simulink model "exp2simulink"  (R2017a)
settings: Solver=ode1  StartTime=0.0  StopTime=27  FixedStep=0.01  RelTol=1e-3
values from neighbouring files (symbols this model uses):
  kkt_4_ASS = 10.^(Gdata(1)/20)    [respostaemfrequencia.m]
  T_4_ASS = 1/abs(pole)    [respostaemfrequencia.m]
undefined symbols (not defined in the file or in its folder): KKt4_ON, T4_ON
libraries: simulink x1
settings Model: Creator=zolubas  LastModifiedBy=zolubas
settings SolverCC: ZeroCrossControl=EnableAll
settings DataIOCC: SaveFormat=Array  SaveOutput=off  TimeSaveName=tsim

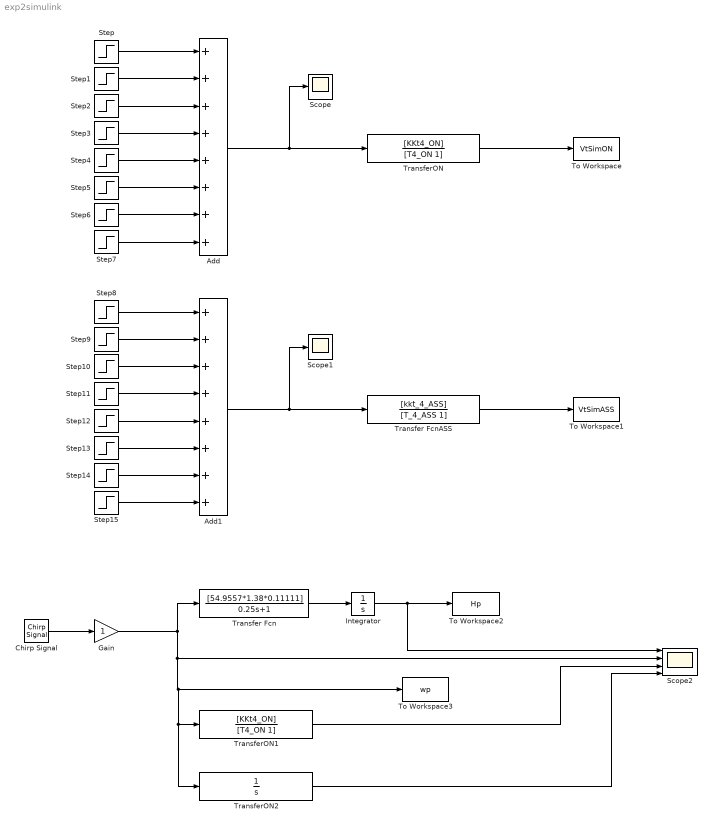
== system exp2simulink ==
  Add : Sum  Inputs=++++++++
  Add1 : Sum  Inputs=++++++++
  Chirp Signal : simulink/Sources/Chirp Signal  f1=0  T=1000  f2=100
  Gain : Gain
  Integrator : Integrator
  Scope : Scope
  Scope1 : Scope
  Scope2 : Scope  NumInputPorts=4
  Step : Step  SampleTime=0
  Step1 : Step  Time=4  After=-2  SampleTime=0
  Step10 : Step  Time=7  After=3  SampleTime=0
  Step11 : Step  Time=10  After=-4  SampleTime=0
  Step12 : Step  Time=13  After=5  SampleTime=0
  Step13 : Step  Time=16  After=-6  SampleTime=0
  Step14 : Step  Time=19  After=7  SampleTime=0
  Step15 : Step  Time=22  After=-8  SampleTime=0
  Step2 : Step  Time=7  After=3  SampleTime=0
  Step3 : Step  Time=10  After=-4  SampleTime=0
  Step4 : Step  Time=13  After=5  SampleTime=0
  Step5 : Step  Time=16  After=-6  SampleTime=0
  Step6 : Step  Time=19  After=7  SampleTime=0
  Step7 : Step  Time=22  After=-8  SampleTime=0
  Step8 : Step  SampleTime=0
  Step9 : Step  Time=4  After=-2  SampleTime=0
  To Workspace : ToWorkspace  VariableName=VtSimON  SampleTime=-1
  To Workspace1 : ToWorkspace  VariableName=VtSimASS  SampleTime=-1
  To Workspace2 : ToWorkspace  VariableName=Hp  SampleTime=-1
  To Workspace3 : ToWorkspace  VariableName=wp  SampleTime=-1
  Transfer Fcn : TransferFcn  Numerator=[54.9557*1.38*0.11111]  Denominator=[0.25 1 ]
  Transfer FcnASS : TransferFcn  Numerator=[kkt_4_ASS]  Denominator=[T_4_ASS 1]
  TransferON : TransferFcn  Numerator=[KKt4_ON]  Denominator=[T4_ON 1]
  TransferON1 : TransferFcn  Numerator=[KKt4_ON]  Denominator=[T4_ON 1]
  TransferON2 : TransferFcn  Denominator=[1 0]
  wires:
  Add/1 -> Scope/1, TransferON/1
  Step/1 -> Add/1
  Step1/1 -> Add/2
  Step2/1 -> Add/3
  Step3/1 -> Add/4
  Step4/1 -> Add/5
  Step5/1 -> Add/6
  Step6/1 -> Add/7
  Step7/1 -> Add/8
  Add1/1 -> Scope1/1, Transfer FcnASS/1
  Step9/1 -> Add1/2
  Step14/1 -> Add1/7
  Step13/1 -> Add1/6
  Step8/1 -> Add1/1
  Step11/1 -> Add1/4
  Step15/1 -> Add1/8
  Step10/1 -> Add1/3
  Step12/1 -> Add1/5
  Transfer FcnASS/1 -> To Workspace1/1
  TransferON/1 -> To Workspace/1
  Chirp Signal/1 -> Gain/1
  Transfer Fcn/1 -> Integrator/1
  TransferON1/1 -> Scope2/3
  Gain/1 -> Transfer Fcn/1, Scope2/2, TransferON2/1, TransferON1/1, To Workspace3/1
  TransferON2/1 -> Scope2/4
  Integrator/1 -> Scope2/1, To Workspace2/1
